simulink model "homework7slx_2015"  (R2015b)
settings: Solver=VariableStepAuto  SolverMode=SingleTasking  StartTime=0.0  StopTime=50.0  RelTol=1e-3
settings Model: Creator=milos  LastModifiedBy=milos
settings DataIOCC: LimitDataPoints=off
settings DebuggingCC: AllowSymbolicDim=on  SFUnexpectedBacktrackingDiag=error  SFNoUnconditionalDefaultTransitionDiag=error
settings ModelReferenceCC: PropagateSignalLabelsOutOfModel=on
settings GRTTargetCC: TargetLangStandard=C99 (ISO)
settings ConfigComp: CovMetricSettings=dwe  CovHtmlReporting=off  CovSaveCumulativeToWorkspaceVar=off  CovSaveSingleToWorkspaceVar=off  CovModelRefEnable=Off  CovExternalEMLEnable=on

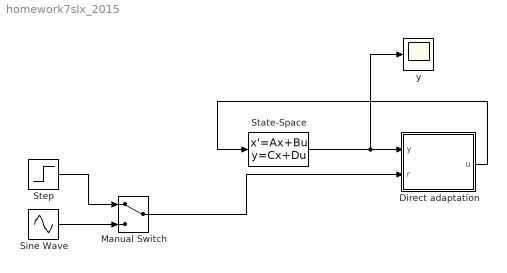
== system homework7slx_2015 ==
  Direct adaptation : Subsystem
  Manual Switch : ManualSwitch
  Sine Wave : Sin  SampleTime=0
  State-Space : StateSpace  A=-3  D=0  X0=0
  Step : Step  SampleTime=0
  y : Scope
  wires:
  State-Space/1 -> y/1, Direct adaptation/1(y)
  Direct adaptation/1(u) -> State-Space/1
  Sine Wave/1 -> Manual Switch/2
  Step/1 -> Manual Switch/1
  Manual Switch/1 -> Direct adaptation/2(r)

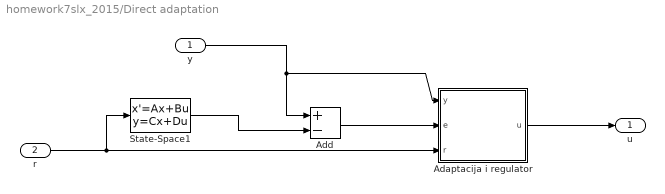
== system homework7slx_2015/Direct adaptation ==
  y : Inport
  r : Inport  Port=2
  Adaptacija i regulator : MATLAB Function  TreatAsAtomicUnit=on
  Add : Sum  Inputs=+-
  State-Space1 : StateSpace  A=-2  B=2  D=0  X0=0
  u : Outport
  wires:
  r/1 -> State-Space1/1, Adaptacija i regulator/3(r)
  Add/1 -> Adaptacija i regulator/2(e)
  y/1 -> Add/1, Adaptacija i regulator/1(y)
  State-Space1/1 -> Add/2
  Adaptacija i regulator/1(u) -> u/1

== matlab function homework7slx_2015/Direct adaptation/Adaptacija i regulator ==
  settings: updateMethod=DISCRETE  sampleTime=T
  data: y input; e input; r input; u output; T parameter
function u = adapAndRegulator(y,e,r,T)
persistent k_p;
persistent kr_p;

if isempty(k_p)
    k_p=0;
    kr_p=0;
end

k=k_p+T*y*e;
kr=kr_p-T*r*e;
k_p=k;
kr_p=kr;

u=-k*y+kr*r;
end
